simulink model "NatersV4_clean"  (R2016a)
settings: Solver=ode5  StartTime=1  StopTime=12*24*3  FixedStep=1  RelTol=1e-3
InitFcn:
  | %open the initialization function as a structure s
  | clear all
  | model = 'NatersV4_clean';
  | s = system_init(model);
  | clear ans
  | 
  | % time vector
  | t=s.t;
  | t_step = t(2)-t(1);
  | time_u = s.time(1);
  | sample_time = s.sample_time;
  | 
  | % declare parameters
  | building = s.building;
  | Text_D = s.Design(1);
  | Tin_D = s.Design(2);
  | Ts_D = s.Design(3);
  | Tr_D = s.Design(4);
  | Qdot_dem = s.Qdot_dem;
  | L_ini= s.L_ini;
  | 
  | Ab_c = s.Ab_c;
  | Bb_c = s.Bb_c;
  | Tin_sp = s.Tin_sp.signals.values;
  | Text = s.Text.signals.values;
  | Rad_90 = s.rad_90.signals.values;
  | 
  | % k parameters for heat pump model
  | K = s.k;
undefined symbols (not defined in the file or in its folder): DiscIntNeverNeededParam
libraries: simulink x17, carnot x2, dspsigops x1
(part 1 of 2)
settings Model: Creator=frederic.amblard  LastModifiedBy=frederic.amblard
settings DataIOCC: ExternalInput=[t, Ab_c, Bb_c, Text, Tin_sp]

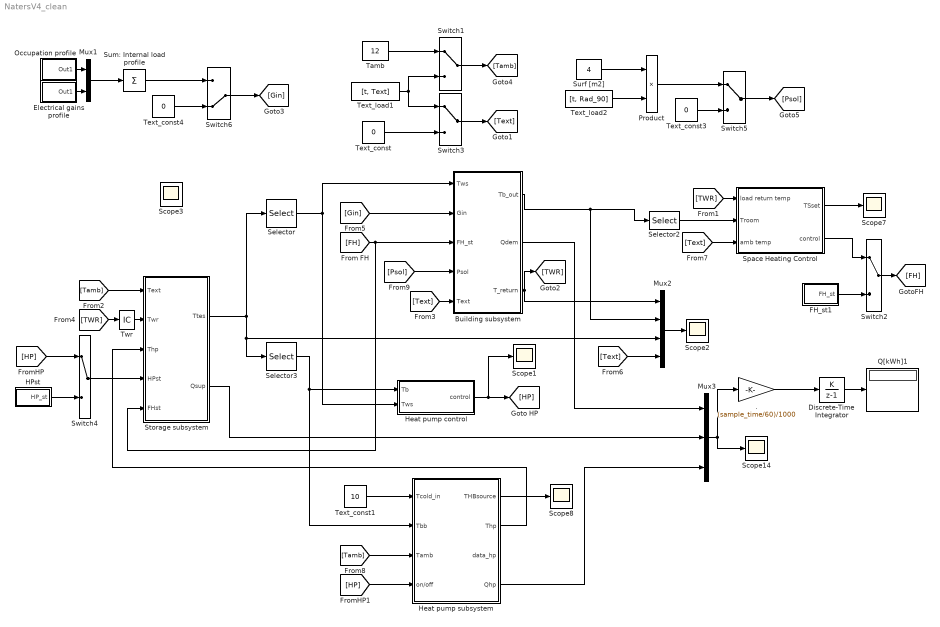
== system NatersV4_clean ==
  . : Gain  Gain=(sample_time/60)/1000  SaturateOnIntegerOverflow=on  OutDataTypeStr=Inherit: Same as input  ParamDataTypeStr=Inherit: Same as input
  Building subsystem : Subsystem
  Discrete-Time Integrator : DiscreteIntegrator  IntegratorMethod=Accumulation: Forward Euler  InitialConditionSetting=State (most efficient)  SampleTime=-1  ICPrevOutput=DiscIntNeverNeededParam  ICPrevScaledInput=DiscIntNeverNeededParam
  Electrical gains profile : Subsystem  mask{period=24*60/sample_time, rep_seq_t=[0 1 6 7 8 9 11 12 13 18 19 20 22 23]*60/sample_time, rep_seq_d=[1 5 1 1 1 2 1 1 4 2 1 2 1 1]*60/sample_time, rep_seq_y=[105 55 392.5 457.5 420 55 250 55 120 170 615 420 442.5 355]*60/sample_time}
      mask prompts: period "Timeperiod in h"; rep_seq_t "Time values in h"; rep_seq_d "Duration in h"; rep_seq_y "Output values"
  FH_st1 : Subsystem  mask{period=24*60/sample_time, rep_seq_t=[0 6 7 8 9 11 12 13 14 15 17 18 20 21 22]*60/sample_time, rep_seq_d=[6 1 1 1 2 1 1 1 1 2 1 2 1 1 2]*60/sample_time, rep_seq_y=[1 1 1 0 0 0 1 1 1 0 0 1 1 1 1]*60/sample_time}
      mask prompts: period "Timeperiod in h"; rep_seq_t "Time values in h"; rep_seq_d "Duration in h"; rep_seq_y "Output values"
  HPst : Subsystem  mask{period=24*60/sample_time, rep_seq_t=[0 6 7 8 9 11 12 13 14 15 17 18 20 21 22]*60/sample_time, rep_seq_d=[6 1 1 1 2 1 1 1 1 2 1 2 1 1 2]*60/sample_time, rep_seq_y=[1 1 1 0 0 0 1 1 1 0 0 1 1 1 1]*60/sample_time}
      mask prompts: period "Timeperiod in h"; rep_seq_t "Time values in h"; rep_seq_d "Duration in h"; rep_seq_y "Output values"
  Heat pump control : Subsystem
  Heat pump subsystem : Subsystem  mask{K=K, caph=80000, capc=50000, cp=4185, DT=4, UA=7, Qdot_D=Qdot_dem}
      mask prompts: K "Param K"; caph "Thermal capacity hot side [J/K]"; capc "Thermal capacity cold side [J/K]"; cp "Heat capacity of water [J/(kg·K)]"; DT "Delta temperature fixed cold side"; UA "Heat loss coefficient [W/K]"; Qdot_D "Design thermal power [W]"
      mask init:
      | mcdot = 1000*Qdot_D/(DT*cp) / 1000; % mass flow [kg/s]
  Mux1 : Mux  Inputs=2
  Mux2 : Mux
  Mux3 : Mux  Inputs=3
  Occupation profile : Subsystem  mask{period=24*60/sample_time, rep_seq_t=[0 6 7 8 9 11 12 13 14 15 17 18 20 21 22]*60/sample_time, rep_seq_d=[6 1 1 1 2 1 1 1 1 2 1 2 1 1 2]*60/sample_time, rep_seq_y=[4 2 3 2 0 1 3 2 1 0 1 2 4 3 4]*60*60/sample_time}
      mask prompts: period "Timeperiod in h"; rep_seq_t "Time values in h"; rep_seq_d "Duration in h"; rep_seq_y "Output values"
  Product : Product
  Q[kWh]1 : Display
  Scope{1..3,7..8,14} (6 alike) : Scope
  Selector : Selector  InputPortWidth=3  IndexOptions=Index vector (dialog)  Indices=[1]  OutputSizes=1
  Selector2 : Selector  InputPortWidth=2  IndexOptions=Index vector (dialog)  Indices=[2]  OutputSizes=1
  Selector3 : Selector  InputPortWidth=3  IndexOptions=Index vector (dialog)  Indices=[3]  OutputSizes=1
  Space Heating Control : Subsystem  mask{Tset=Tin_D, Tsetn=Tin_D, Q_LOC=Qdot_dem, Td_in=Ts_D, Td_out=Tr_D, Tambd=Text_D, n_rad=1.1}
      mask prompts: Tset "desired room day Temperature [°C]"; Tsetn "desired room night Temperature [°C]"; Q_LOC "design heat load [W]"; Td_in "design inlet temperature of the heating system [°C]"; Td_out "design outlet temperature of the heating system [°C]"; Tambd "design outdoor temperature"; n_rad "radiatior exponent"
      mask init:
      | dTd = 0.5*(Td_in + Td_out) - Tset;
      | dTdn = 0.5*(Td_in + Td_out) - Tsetn;
  Storage subsystem : Subsystem
  Sum: Internal load profile : Sum  Inputs=+
  Surf [m2] : Constant  Value=4
  Switch{1..5} (5 alike) : ManualSwitch
  Switch6 : ManualSwitch  CurrentSetting=0
  Tamb : Constant  Value=12
  Text_const : Constant  Value=0
  Text_const1 : Constant  Value=10
  Text_const3 : Constant  Value=0
  Text_const4 : Constant  Value=0
  Text_load1 : FromWorkspace  Tag=Tin_sp  Description=Temperature signal of the room  VariableName=[t, Text]  SampleTime=1  Interpolate=off  OutputAfterFinalValue=Setting to zero
  Text_load2 : FromWorkspace  Tag=Tin_sp  Description=Temperature signal of the room  VariableName=[t, Rad_90]  SampleTime=1  Interpolate=off  OutputAfterFinalValue=Setting to zero
  Twr : InitialCondition  Value=Tr_D
  wires:
  Text_load1/1 -> Switch1/2, Switch3/1
  Text_const/1 -> Switch3/2
  Switch3/1 -> [Text]
  [Tamb] -> Storage subsystem/1(Text)
  Storage subsystem/1(Ttes) -> Selector/1, Selector3/1, Mux2/3
  Occupation profile/1(Out1) -> Mux1/1
  Electrical gains profile/1(Out1) -> Mux1/2
  Mux1/1 -> Sum: Internal load profile/1
  Sum: Internal load profile/1 -> Switch6/1
  Building subsystem/1(Tb_out) -> Mux2/2, Selector2/1
  Building subsystem/3(T_return) -> Mux2/1, [TWR]
  [TWR] -> Twr/1
  Twr/1 -> Storage subsystem/2(Twr)
  [Gin] -> Building subsystem/2(Gin)
  Text_load2/1 -> Product/2
  Mux2/1 -> Scope2/1
  HPst/1(HP_st) -> Switch4/2
  [Text] -> Mux2/4
  Tamb/1 -> Switch1/1
  Switch1/1 -> [Tamb]
  [FH] -> Storage subsystem/5(FHst), Building subsystem/3(FH_st)
  Selector2/1 -> Space Heating Control/2(Troom)
  [Text] -> Space Heating Control/3(amb temp)
  Space Heating Control/1(TSset) -> Scope7/1
  Space Heating Control/2(control) -> Switch2/1
  FH_st1/1(FH_st) -> Switch2/2
  Switch2/1 -> [FH]
  Switch4/1 -> Storage subsystem/4(HPst)
  [HP] -> Switch4/1
  Selector3/1 -> Heat pump subsystem/2(Tbb), Heat pump control/1(Tb)
  [Tamb] -> Heat pump subsystem/3(Tamb)
  [HP] -> Heat pump subsystem/4(on/off)
  Heat pump subsystem/1(THBsource) -> Scope8/1
  Heat pump subsystem/2(Thp) -> Storage subsystem/3(Thp)
  Text_const1/1 -> Heat pump subsystem/1(Tcold_in)
  Surf [m2]/1 -> Product/1
  Product/1 -> Switch5/1
  [Psol] -> Building subsystem/4(Psol)
  Storage subsystem/2(Qsup) -> Mux3/2
  Building subsystem/2(Qdem) -> Mux3/1
  Selector/1 -> Heat pump control/2(Tws), Building subsystem/1(Tws)
  Mux3/1 -> Scope14/1, ./1
  Discrete-Time Integrator/1 -> Q[kWh]1/1
  ./1 -> Discrete-Time Integrator/1
  Text_const3/1 -> Switch5/2
  Switch5/1 -> [Psol]
  Text_const4/1 -> Switch6/2
  Switch6/1 -> [Gin]
  Heat pump subsystem/4(Qhp) -> Mux3/3
  [Text] -> Building subsystem/5(Text)
  Heat pump control/1(control) -> Scope1/1, [HP]
  [TWR] -> Space Heating Control/1(load return temp)

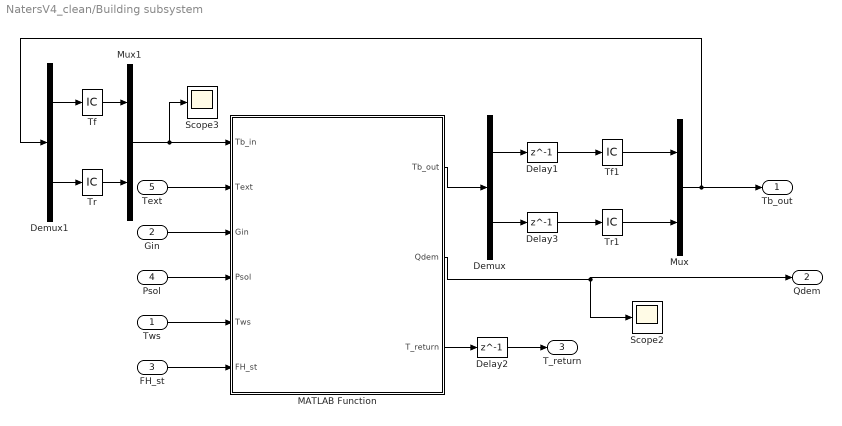
== system NatersV4_clean/Building subsystem ==
  Tws : Inport
  Gin : Inport  Port=2
  FH_st : Inport  Port=3
  Psol : Inport  Port=4
  Text : Inport  Port=5
  Delay1 : Delay  DelayLength=1  InitialCondition=0
  Delay2 : Delay  DelayLength=1  InitialCondition=0
  Delay3 : Delay  DelayLength=1  InitialCondition=0
  Demux : Demux  Outputs=2
  Demux1 : Demux  Outputs=2
  MATLAB Function : MATLAB Function  TreatAsAtomicUnit=on  mask{t_step=t_step, time_u=time_u}
      mask prompts: t_step "time_sample"; time_u "time_unit"
  Mux : Mux  Inputs=2
  Mux1 : Mux  Inputs=2
  Scope2 : Scope
  Scope3 : Scope
  Tf : InitialCondition  Value=22
  Tf1 : InitialCondition  Value=22
  Tr : InitialCondition  Value=20
  Tr1 : InitialCondition  Value=20
  Tb_out : Outport
  Qdem : Outport  Port=2
  T_return : Outport  Port=3
  wires:
  MATLAB Function/1(Tb_out) -> Demux/1
  Delay1/1 -> Tf1/1
  Delay3/1 -> Tr1/1
  Demux/1 -> Delay1/1
  Demux/2 -> Delay3/1
  Mux/1 -> Demux1/1, Tb_out/1
  Tr/1 -> Mux1/2
  Demux1/2 -> Tr/1
  Demux1/1 -> Tf/1
  Tf/1 -> Mux1/1
  Mux1/1 -> Scope3/1, MATLAB Function/1(Tb_in)
  FH_st/1 -> MATLAB Function/6(FH_st)
  Gin/1 -> MATLAB Function/3(Gin)
  Psol/1 -> MATLAB Function/4(Psol)
  MATLAB Function/2(Qdem) -> Scope2/1, Qdem/1
  Tws/1 -> MATLAB Function/5(Tws)
  Text/1 -> MATLAB Function/2(Text)
  Tf1/1 -> Mux/1
  Tr1/1 -> Mux/2
  MATLAB Function/3(T_return) -> Delay2/1
  Delay2/1 -> T_return/1

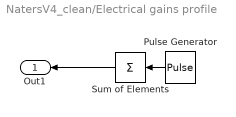
== system NatersV4_clean/Electrical gains profile ==
  Pulse Generator : DiscretePulseGenerator  PulseType=Time based  Amplitude=rep_seq_y  Period=period  PulseWidth=rep_seq_d*100/period  PhaseDelay=rep_seq_t
  Sum of Elements : Sum  Inputs=+
  Out1 : Outport
  wires:
  Sum of Elements/1 -> Out1/1
  Pulse Generator/1 -> Sum of Elements/1

== system NatersV4_clean/FH_st1 ==
  Pulse Generator : DiscretePulseGenerator  PulseType=Time based  Amplitude=rep_seq_y  Period=period  PulseWidth=rep_seq_d*100/period  PhaseDelay=rep_seq_t
  Sum of Elements : Sum  Inputs=+
  FH_st : Outport
  wires:
  Sum of Elements/1 -> FH_st/1
  Pulse Generator/1 -> Sum of Elements/1

== system NatersV4_clean/HPst ==
  Pulse Generator : DiscretePulseGenerator  PulseType=Time based  Amplitude=rep_seq_y  Period=period  PulseWidth=rep_seq_d*100/period  PhaseDelay=rep_seq_t
  Sum of Elements : Sum  Inputs=+
  HP_st : Outport
  wires:
  Sum of Elements/1 -> HP_st/1
  Pulse Generator/1 -> Sum of Elements/1

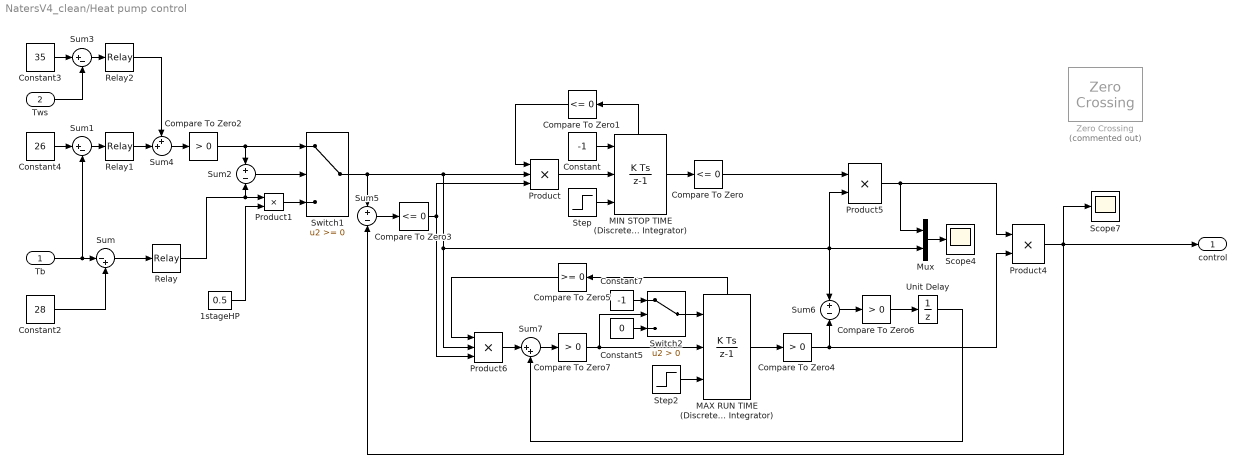
== system NatersV4_clean/Heat pump control ==
  Tb : Inport
  Tws : Inport  Port=2
  1stageHP : Constant  Value=0.5
  Compare To Zero : simulink/Logic and Bit Operations/Compare To Zero  relop=<=  OutDataTypeStr=uint8
  Compare To Zero1 : simulink/Logic and Bit Operations/Compare To Zero  relop=<=  OutDataTypeStr=uint8
  Compare To Zero2 : simulink/Logic and Bit Operations/Compare To Zero  relop=>  OutDataTypeStr=boolean
  Compare To Zero3 : simulink/Logic and Bit Operations/Compare To Zero  relop=<=  OutDataTypeStr=uint8
  Compare To Zero4 : simulink/Logic and Bit Operations/Compare To Zero  relop=>  OutDataTypeStr=uint8
  Compare To Zero5 : simulink/Logic and Bit Operations/Compare To Zero  relop=>=  OutDataTypeStr=uint8
  Compare To Zero6 : simulink/Logic and Bit Operations/Compare To Zero  relop=>  OutDataTypeStr=uint8
  Compare To Zero7 : simulink/Logic and Bit Operations/Compare To Zero  relop=>  OutDataTypeStr=uint8
  Constant : Constant  Value=-1
  Constant2 : Constant  Value=28
  Constant3 : Constant  Value=35
  Constant4 : Constant  Value=26
  Constant5 : Constant  Value=0  SampleTime=-1
  Constant7 : Constant  Value=-1  SampleTime=-1
  MAX RUN TIME (Discrete-Time Integrator) : DiscreteIntegrator  ExternalReset=falling  InitialConditionSource=external  InitialConditionSetting=State (most efficient)  SampleTime=-1  LowerSaturationLimit=0  ShowStatePort=on  IgnoreLimit=on  ICPrevOutput=DiscIntNeverNeededParam  ICPrevScaledInput=DiscIntNeverNeededParam
  MIN STOP TIME (Discrete-Time Integrator) : DiscreteIntegrator  ExternalReset=falling  InitialConditionSource=external  InitialConditionSetting=State (most efficient)  SampleTime=-1  LimitOutput=on  LowerSaturationLimit=0  ShowStatePort=on  ICPrevOutput=DiscIntNeverNeededParam  ICPrevScaledInput=DiscIntNeverNeededParam
  Mux : Mux  Inputs=2
  Product : Product  Inputs=3  RndMeth=Zero
  Product1 : Product  RndMeth=Zero
  Product4 : Product  RndMeth=Zero
  Product5 : Product  RndMeth=Zero
  Product6 : Product  Inputs=3  RndMeth=Zero
  Relay : Relay  OnSwitchValue=1  OffSwitchValue=-6
  Relay1 : Relay  OnSwitchValue=1  OffSwitchValue=-2
  Relay2 : Relay  OnSwitchValue=1  OffSwitchValue=-6
  Scope4 : Scope
  Scope7 : Scope
  Step : Step  After=15/sample_time  SampleTime=1
  Step2 : Step  After=300/sample_time  SampleTime=1  VectorParams1D=off
  Sum : Sum  Inputs=|-+
  Sum1 : Sum  Inputs=|+-
  Sum2 : Sum  Inputs=+|-
  Sum3 : Sum  Inputs=|+-
  Sum4 : Sum  Inputs=++|
  Sum5 : Sum  Inputs=+|-
  Sum6 : Sum  Inputs=+|-
  Sum7 : Sum  Inputs=|++
  Switch1 : Switch
  Switch2 : Switch  Criteria=u2 > Threshold
  Unit Delay : UnitDelay  SampleTime=-1
  Zero Crossing : dspsigops/Zero Crossing  Commented=on  InputProcessing=Columns as channels (frame based)
  control : Outport
  wires:
  Tb/1 -> Sum/1, Sum1/2
  Constant2/1 -> Sum/2
  Sum/1 -> Relay/1
  Product/1 -> MIN STOP TIME (Discrete-Time Integrator)/2
  MIN STOP TIME (Discrete-Time Integrator)/State -> Compare To Zero1/1
  Compare To Zero1/1 -> Product/1
  Constant/1 -> MIN STOP TIME (Discrete-Time Integrator)/1
  Step/1 -> MIN STOP TIME (Discrete-Time Integrator)/3
  MIN STOP TIME (Discrete-Time Integrator)/1 -> Compare To Zero/1
  Mux/1 -> Scope4/1
  Compare To Zero/1 -> Product5/1
  Product5/1 -> Mux/1, Product4/1
  MAX RUN TIME (Discrete-Time Integrator)/State -> Compare To Zero5/1
  Step2/1 -> MAX RUN TIME (Discrete-Time Integrator)/3
  Relay/1 -> Product1/1, Sum2/2
  1stageHP/1 -> Product1/2
  Constant4/1 -> Sum1/1
  Sum1/1 -> Relay1/1
  Sum4/1 -> Compare To Zero2/1
  Product1/1 -> Switch1/3
  Sum2/1 -> Switch1/2
  Constant3/1 -> Sum3/1
  Tws/1 -> Sum3/2
  Sum3/1 -> Relay2/1
  Relay2/1 -> Sum4/1
  Relay1/1 -> Sum4/2
  Product4/1 -> control/1, Scope7/1, Sum5/2
  Compare To Zero2/1 -> Switch1/1, Sum2/1
  Switch1/1 -> Product/2, Product6/2, Product5/2, Mux/2, Sum6/1, Sum5/1
  Sum5/1 -> Compare To Zero3/1
  Sum6/1 -> Compare To Zero6/1
  Product6/1 -> Sum7/1
  Compare To Zero6/1 -> Unit Delay/1
  Compare To Zero4/1 -> Sum6/2, Product4/2
  Compare To Zero3/1 -> Product/3, Product6/3
  Sum7/1 -> Compare To Zero7/1
  Compare To Zero7/1 -> Switch2/2, MAX RUN TIME (Discrete-Time Integrator)/2
  Unit Delay/1 -> Sum7/2
  Constant7/1 -> Switch2/1
  Compare To Zero5/1 -> Product6/1
  MAX RUN TIME (Discrete-Time Integrator)/1 -> Compare To Zero4/1
  Switch2/1 -> MAX RUN TIME (Discrete-Time Integrator)/1
  Constant5/1 -> Switch2/3

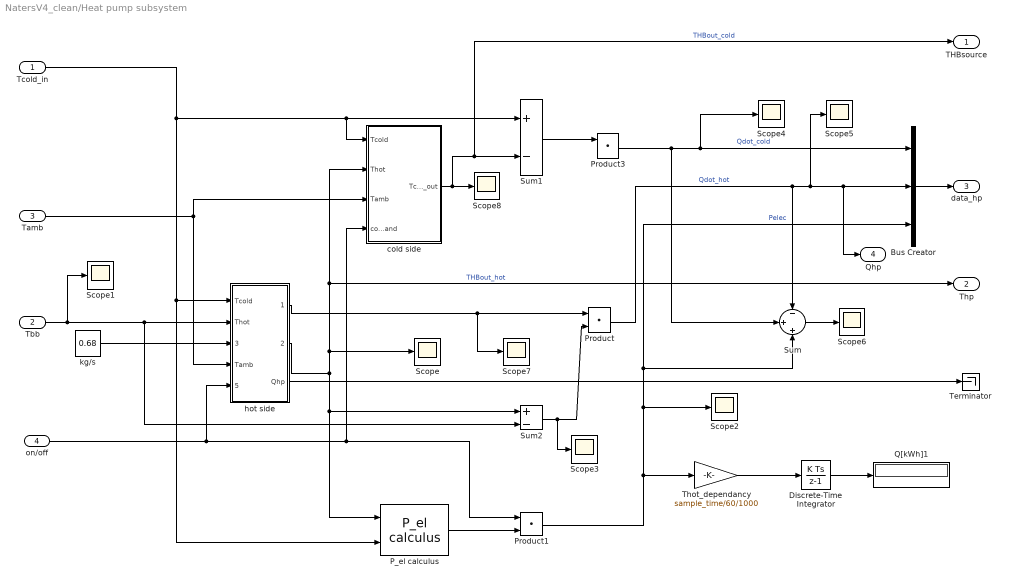
== system NatersV4_clean/Heat pump subsystem ==
  Tcold_in : Inport
  Tbb : Inport  Port=2
  Tamb : Inport  Port=3
  on/off : Inport  Port=4
  Bus Creator : BusCreator  Inputs=3
  Discrete-Time Integrator : DiscreteIntegrator  InitialConditionSetting=State (most efficient)  SampleTime=-1  ICPrevOutput=DiscIntNeverNeededParam  ICPrevScaledInput=DiscIntNeverNeededParam
  P_el calculus : carnot/Basic/Thermal_Models/HeatPump_basic/P_el calculus
  Product : DotProduct  InputSameDT=on  OutDataTypeStr=Inherit: Inherit via internal rule
  Product1 : DotProduct  InputSameDT=on  OutDataTypeStr=Inherit: Inherit via internal rule
  Product3 : DotProduct  InputSameDT=on  OutDataTypeStr=Inherit: Inherit via internal rule
  Q[kWh]1 : Display
  Scope{,1..8} (9 alike) : Scope
  Sum : Sum  Inputs=-|+|+
  Sum1 : Sum  Inputs=+-  SaturateOnIntegerOverflow=on  InputSameDT=on  OutDataTypeStr=Inherit: Same as first input
  Sum2 : Sum  Inputs=+-  SaturateOnIntegerOverflow=on  InputSameDT=on  OutDataTypeStr=Inherit: Same as first input
  Terminator : Terminator
  Thot_dependancy : Gain  Gain=sample_time/60/1000  SaturateOnIntegerOverflow=on  OutDataTypeStr=Inherit: Same as input  ParamDataTypeStr=Inherit: Same as input
  cold side : Subsystem
  hot side : Subsystem
  kg/s : Constant  Value=0.68
  THBsource : Outport
  Thp : Outport  Port=2
  data_hp : Outport  Port=3
  Qhp : Outport  Port=4
  wires:
  Bus Creator/1 -> data_hp/1
  cold side/1(Tcold_out) -> THBsource/1, Sum1/2, Scope8/1  "THBout_cold"
  hot side/2(Thot_out) -> cold side/2(Thot), Thp/1, Scope/1, P_el calculus/1, Sum2/1  "THBout_hot"
  Tamb/1 -> cold side/3(Tamb), hot side/4(Tamb)
  Tbb/1 -> Scope1/1, hot side/2(Thot), Sum2/2
  hot side/1(mdot*cp) -> Scope7/1, Product/1
  Sum2/1 -> Scope3/1, Product/2
  Tcold_in/1 -> hot side/1(Tcold), P_el calculus/2, cold side/1(Tcold), Sum1/1
  P_el calculus/1 -> Product1/2
  Product1/1 -> Thot_dependancy/1, Scope2/1, Sum/3, Bus Creator/3  "Pelec"
  on/off/1 -> hot side/5(command), cold side/4(command), Product1/1
  Sum1/1 -> Product3/1
  Product3/1 -> Sum/2, Scope4/1, Bus Creator/1  "Qdot_cold"
  Product/1 -> Sum/1, Scope5/1, Qhp/1, Bus Creator/2  "Qdot_hot"
  kg/s/1 -> hot side/3(mdot_hot)
  Discrete-Time Integrator/1 -> Q[kWh]1/1
  Thot_dependancy/1 -> Discrete-Time Integrator/1
  Sum/1 -> Scope6/1
  hot side/3(Qhp) -> Terminator/1

== system NatersV4_clean/Occupation profile ==
  Pulse Generator : DiscretePulseGenerator  PulseType=Time based  Amplitude=rep_seq_y  Period=period  PulseWidth=rep_seq_d*100/period  PhaseDelay=rep_seq_t
  Sum of Elements : Sum  Inputs=+
  Out1 : Outport
  wires:
  Sum of Elements/1 -> Out1/1
  Pulse Generator/1 -> Sum of Elements/1

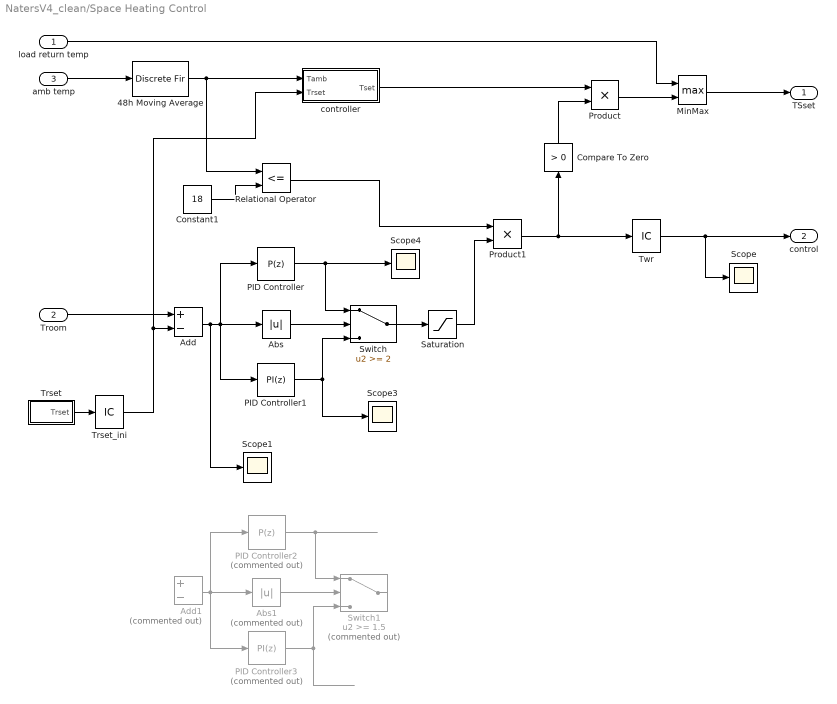
== system NatersV4_clean/Space Heating Control ==
  load return temp : Inport
  Troom : Inport  Port=2
  amb temp : Inport  Port=3
  48h Moving Average : DiscreteFir  Coefficients=ones(1,60/sample_time*24)*(1/((60/sample_time)*24))  SampleTime=1  AccumDataTypeStr=Inherit: Same as product output  RndMeth=Nearest
  Abs : Abs
  Abs1 : Abs  Commented=on
  Add : Sum  Inputs=+-
  Add1 : Sum  Commented=on  Inputs=+-
  Compare To Zero : simulink/Logic and Bit Operations/Compare To Zero  relop=>  OutDataTypeStr=boolean
  Constant1 : Constant  Value=18
  MinMax : MinMax  Function=max  Inputs=2
  PID Controller : simulink/Continuous/PID Controller  Controller=P  TimeDomain=Discrete-time  SampleTime=-1  IntegratorMethod=Forward Euler  FilterMethod=Forward Euler  Form=Parallel  UseFilter=on  ControllerParametersSource=internal  P=-0.6  I=1  D=0  N=100  InitialConditionSource=internal  InitialConditionForIntegrator=0  InitialConditionForFilter=0  ExternalReset=none  ZeroCross=off  LimitOutput=on  UpperSaturationLimit=1  LowerSaturationLimit=0  LinearizeAsGain=off  AntiWindupMode=none  Kb=1  TrackingMode=off  Kt=1  PParamMin=[]  PParamMax=[]  IParamMin=[]  IParamMax=[]  DParamMin=[]  DParamMax=[]  NParamMin=[]  NParamMax=[]  KbParamMin=[]  KbParamMax=[]  KtParamMin=[]  KtParamMax=[]  POutMin=[]  POutMax=[]  IOutMin=[]  IOutMax=[]  DOutMin=[]  DOutMax=[]  NOutMin=[]  NOutMax=[]  KbOutMin=[]  KbOutMax=[]  KtOutMin=[]  KtOutMax=[]  IntegratorOutMin=[]  IntegratorOutMax=[]  FilterOutMin=[]  FilterOutMax=[]  SumOutMin=[]  SumOutMax=[]  SumI1OutMin=[]  SumI1OutMax=[]  SumI2OutMin=[]  SumI2OutMax=[]  SumI3OutMin=[]  SumI3OutMax=[]  SumDOutMin=[]  SumDOutMax=[]  SaturationOutMin=[]  SaturationOutMax=[]  IntegratorContinuousStateAttributes=''  IntegratorStateMustResolveToSignalObject=off  IntegratorRTWStateStorageClass=Auto  FilterContinuousStateAttributes=''  FilterStateMustResolveToSignalObject=off  FilterRTWStateStorageClass=Auto  DifferentiatorICPrevScaledInput=0  DifferentiatorOutMin=[]  DifferentiatorOutMax=[]
  PID Controller1 : simulink/Continuous/PID Controller  Controller=PI  TimeDomain=Discrete-time  SampleTime=-1  IntegratorMethod=Trapezoidal  FilterMethod=Forward Euler  Form=Parallel  UseFilter=on  ControllerParametersSource=internal  P=-8  I=-0.8/(60*sample_time)  D=0.001  N=100  InitialConditionSource=internal  InitialConditionForIntegrator=0  InitialConditionForFilter=0  ExternalReset=none  LimitOutput=on  UpperSaturationLimit=1  LowerSaturationLimit=0  LinearizeAsGain=off  AntiWindupMode=back-calculation  Kb=1  TrackingMode=off  Kt=1  PParamMin=[]  PParamMax=[]  IParamMin=[]  IParamMax=[]  DParamMin=[]  DParamMax=[]  NParamMin=[]  NParamMax=[]  KbParamMin=[]  KbParamMax=[]  KtParamMin=[]  KtParamMax=[]  POutMin=[]  POutMax=[]  IOutMin=[]  IOutMax=[]  DOutMin=[]  DOutMax=[]  NOutMin=[]  NOutMax=[]  KbOutMin=[]  KbOutMax=[]  KtOutMin=[]  KtOutMax=[]  IntegratorOutMin=[]  IntegratorOutMax=[]  FilterOutMin=[]  FilterOutMax=[]  SumOutMin=[]  SumOutMax=[]  SumI1OutMin=[]  SumI1OutMax=[]  SumI2OutMin=[]  SumI2OutMax=[]  SumI3OutMin=[]  SumI3OutMax=[]  SumDOutMin=[]  SumDOutMax=[]  SaturationOutMin=[]  SaturationOutMax=[]  IntegratorContinuousStateAttributes=''  IntegratorStateMustResolveToSignalObject=off  IntegratorRTWStateStorageClass=Auto  FilterContinuousStateAttributes=''  FilterStateMustResolveToSignalObject=off  FilterRTWStateStorageClass=Auto  DifferentiatorICPrevScaledInput=0  DifferentiatorOutMin=[]  DifferentiatorOutMax=[]
  PID Controller2 : simulink/Continuous/PID Controller  Commented=on  Controller=P  TimeDomain=Discrete-time  SampleTime=-1  IntegratorMethod=Forward Euler  FilterMethod=Forward Euler  Form=Parallel  UseFilter=on  ControllerParametersSource=internal  P=-0.5  I=1  D=0  N=100  InitialConditionSource=internal  InitialConditionForIntegrator=0  InitialConditionForFilter=0  ExternalReset=none  ZeroCross=off  LimitOutput=on  UpperSaturationLimit=1  LowerSaturationLimit=0  LinearizeAsGain=off  AntiWindupMode=none  Kb=1  TrackingMode=off  Kt=1  PParamMin=[]  PParamMax=[]  IParamMin=[]  IParamMax=[]  DParamMin=[]  DParamMax=[]  NParamMin=[]  NParamMax=[]  KbParamMin=[]  KbParamMax=[]  KtParamMin=[]  KtParamMax=[]  POutMin=[]  POutMax=[]  IOutMin=[]  IOutMax=[]  DOutMin=[]  DOutMax=[]  NOutMin=[]  NOutMax=[]  KbOutMin=[]  KbOutMax=[]  KtOutMin=[]  KtOutMax=[]  IntegratorOutMin=[]  IntegratorOutMax=[]  FilterOutMin=[]  FilterOutMax=[]  SumOutMin=[]  SumOutMax=[]  SumI1OutMin=[]  SumI1OutMax=[]  SumI2OutMin=[]  SumI2OutMax=[]  SumI3OutMin=[]  SumI3OutMax=[]  SumDOutMin=[]  SumDOutMax=[]  SaturationOutMin=[]  SaturationOutMax=[]  IntegratorContinuousStateAttributes=''  IntegratorStateMustResolveToSignalObject=off  IntegratorRTWStateStorageClass=Auto  FilterContinuousStateAttributes=''  FilterStateMustResolveToSignalObject=off  FilterRTWStateStorageClass=Auto  DifferentiatorICPrevScaledInput=0  DifferentiatorOutMin=[]  DifferentiatorOutMax=[]
  PID Controller3 : simulink/Continuous/PID Controller  Commented=on  Controller=PI  TimeDomain=Discrete-time  SampleTime=-1  IntegratorMethod=Backward Euler  FilterMethod=Forward Euler  Form=Parallel  UseFilter=on  ControllerParametersSource=internal  P=-0.6  I=-0.05/(60*sample_time)  D=0.001  N=100  InitialConditionSource=internal  InitialConditionForIntegrator=0  InitialConditionForFilter=0  ExternalReset=none  ZeroCross=off  LimitOutput=on  UpperSaturationLimit=1  LowerSaturationLimit=0  LinearizeAsGain=off  AntiWindupMode=back-calculation  Kb=1  TrackingMode=off  Kt=1  PParamMin=[]  PParamMax=[]  IParamMin=[]  IParamMax=[]  DParamMin=[]  DParamMax=[]  NParamMin=[]  NParamMax=[]  KbParamMin=[]  KbParamMax=[]  KtParamMin=[]  KtParamMax=[]  POutMin=[]  POutMax=[]  IOutMin=[]  IOutMax=[]  DOutMin=[]  DOutMax=[]  NOutMin=[]  NOutMax=[]  KbOutMin=[]  KbOutMax=[]  KtOutMin=[]  KtOutMax=[]  IntegratorOutMin=[]  IntegratorOutMax=[]  FilterOutMin=[]  FilterOutMax=[]  SumOutMin=[]  SumOutMax=[]  SumI1OutMin=[]  SumI1OutMax=[]  SumI2OutMin=[]  SumI2OutMax=[]  SumI3OutMin=[]  SumI3OutMax=[]  SumDOutMin=[]  SumDOutMax=[]  SaturationOutMin=[]  SaturationOutMax=[]  IntegratorContinuousStateAttributes=''  IntegratorStateMustResolveToSignalObject=off  IntegratorRTWStateStorageClass=Auto  FilterContinuousStateAttributes=''  FilterStateMustResolveToSignalObject=off  FilterRTWStateStorageClass=Auto  DifferentiatorICPrevScaledInput=0  DifferentiatorOutMin=[]  DifferentiatorOutMax=[]
  Product : Product
  Product1 : Product
  Relational Operator : RelationalOperator  Operator=<=  OutDataTypeStr=boolean
  Saturation : Saturate  UpperLimit=1  LowerLimit=0  LinearizeAsGain=off  ZeroCross=off
  Scope{,1,3..4} (4 alike) : Scope
  Switch : Switch  Threshold=2
  Switch1 : Switch  Commented=on  Threshold=1.5
  Trset : Subsystem  mask{period=24*60/sample_time, rep_seq_t=[0 7 21]*60/sample_time, rep_seq_d=[7 14 3]*60/sample_time, rep_seq_y=[Tsetn Tset Tsetn]}
      mask prompts: period "Timeperiod in h"; rep_seq_t "Time values in h"; rep_seq_d "Duration in h"; rep_seq_y "Output values"
  Trset_ini : InitialCondition  Value=19.9
  Twr : InitialCondition  Value=L_ini
  controller : Subsystem
  TSset : Outport
  control : Outport  Port=2
  wires:
  amb temp/1 -> 48h Moving Average/1
  Constant1/1 -> Relational Operator/2
  Troom/1 -> Add/1
  Add/1 -> Scope1/1, PID Controller/1, PID Controller1/1, Abs/1
  Abs/1 -> Switch/2
  PID Controller/1 -> Scope4/1, Switch/1
  PID Controller1/1 -> Switch/3, Scope3/1
  Switch/1 -> Saturation/1
  Saturation/1 -> Product1/2
  Product/1 -> MinMax/2
  load return temp/1 -> MinMax/1
  Compare To Zero/1 -> Product/2
  48h Moving Average/1 -> Relational Operator/1, controller/1(Tamb)
  controller/1(Tset) -> Product/1
  Relational Operator/1 -> Product1/1
  MinMax/1 -> TSset/1
  Trset/1(Trset) -> Trset_ini/1
  Product1/1 -> Twr/1, Compare To Zero/1
  Add1/1 -> PID Controller2/1, PID Controller3/1, Abs1/1
  Abs1/1 -> Switch1/2
  PID Controller2/1 -> Switch1/1
  PID Controller3/1 -> Switch1/3
  Twr/1 -> Scope/1, control/1
  Trset_ini/1 -> controller/2(Trset), Add/2

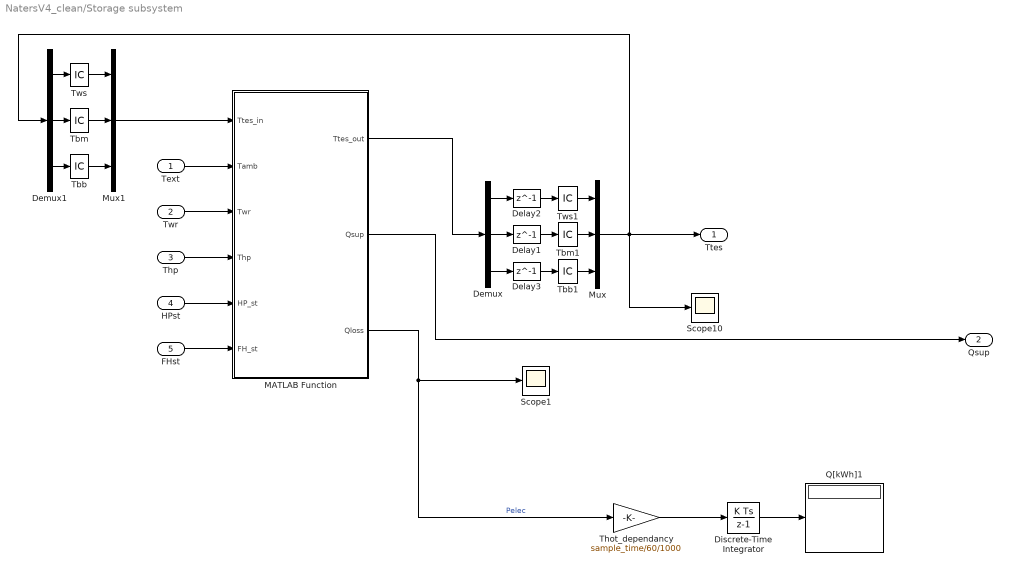
== system NatersV4_clean/Storage subsystem ==
  Text : Inport
  Twr : Inport  Port=2
  Thp : Inport  Port=3
  HPst : Inport  Port=4
  FHst : Inport  Port=5
  Delay1 : Delay  DelayLength=1  InitialCondition=0
  Delay2 : Delay  DelayLength=1  InitialCondition=0
  Delay3 : Delay  DelayLength=1  InitialCondition=0
  Demux : Demux  Outputs=3
  Demux1 : Demux  Outputs=3
  Discrete-Time Integrator : DiscreteIntegrator  InitialConditionSetting=State (most efficient)  SampleTime=-1  ICPrevOutput=DiscIntNeverNeededParam  ICPrevScaledInput=DiscIntNeverNeededParam
  MATLAB Function : MATLAB Function  TreatAsAtomicUnit=on  mask{t_step=t_step, time_u=time_u}
      mask prompts: t_step "sampling_time"; time_u "time_unit"
  Mux : Mux  Inputs=3
  Mux1 : Mux  Inputs=3
  Q[kWh]1 : Display
  Scope1 : Scope
  Scope10 : Scope
  Tbb : InitialCondition  Value=28
  Tbb1 : InitialCondition  Value=28
  Tbm : InitialCondition  Value=31
  Tbm1 : InitialCondition  Value=31
  Thot_dependancy : Gain  Gain=sample_time/60/1000  SaturateOnIntegerOverflow=on  OutDataTypeStr=Inherit: Same as input  ParamDataTypeStr=Inherit: Same as input
  Tws : InitialCondition  Value=35
  Tws1 : InitialCondition  Value=35
  Ttes : Outport
  Qsup : Outport  Port=2
  wires:
  MATLAB Function/1(Ttes_out) -> Demux/1
  Delay2/1 -> Tws1/1
  Delay1/1 -> Tbm1/1
  Text/1 -> MATLAB Function/2(Tamb)
  HPst/1 -> MATLAB Function/5(HP_st)
  FHst/1 -> MATLAB Function/6(FH_st)
  Demux/1 -> Delay2/1
  Demux/2 -> Delay1/1
  Demux1/2 -> Tbm/1
  Tbm/1 -> Mux1/2
  Demux1/1 -> Tws/1
  Tws/1 -> Mux1/1
  Mux1/1 -> MATLAB Function/1(Ttes_in)
  Thp/1 -> MATLAB Function/4(Thp)
  MATLAB Function/2(Qsup) -> Qsup/1
  Twr/1 -> MATLAB Function/3(Twr)
  Discrete-Time Integrator/1 -> Q[kWh]1/1
  Thot_dependancy/1 -> Discrete-Time Integrator/1
  MATLAB Function/3(Qloss) -> Scope1/1, Thot_dependancy/1  "Pelec"
  Demux/3 -> Delay3/1
  Delay3/1 -> Tbb1/1
  Demux1/3 -> Tbb/1
  Tbb/1 -> Mux1/3
  Mux/1 -> Ttes/1, Scope10/1, Demux1/1
  Tws1/1 -> Mux/1
  Tbm1/1 -> Mux/2
  Tbb1/1 -> Mux/3

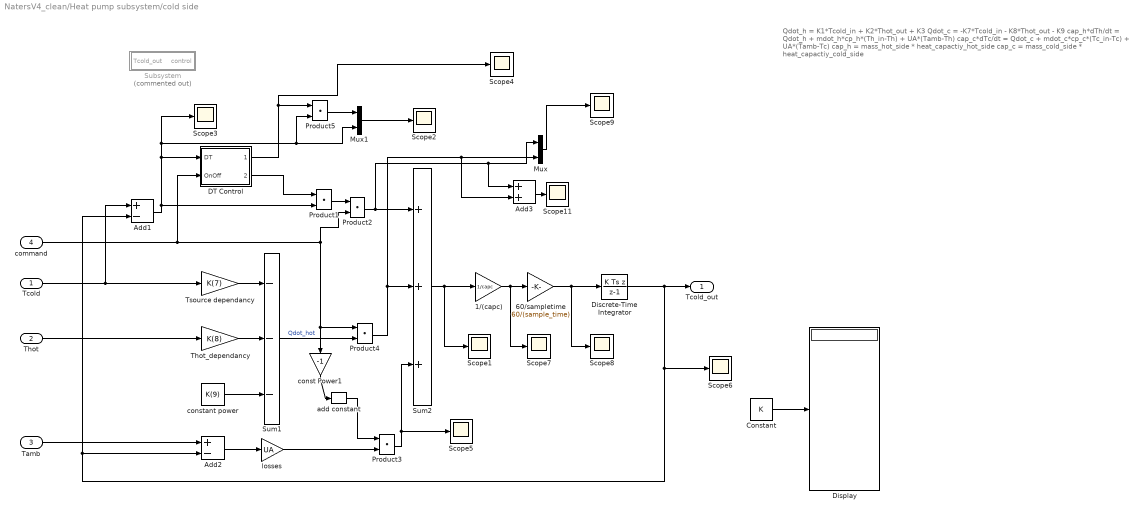
== system NatersV4_clean/Heat pump subsystem/cold side ==
  note: Qdot_h = K1*Tcold_in + K2*Thot_out + K3
      |
      | Qdot_c = -K7*Tcold_in - K8*Thot_out - K9
      |
      | cap_h*dTh/dt = Qdot_h + mdot_h*cp_h*(Th_in-Th) + UA*(Tamb-Th)
      |
      | cap_c*dTc/dt = Qdot_c + mdot_c*cp_c*(Tc_in-Tc) + UA*(Tamb-Tc)
      |
      | cap_h = mass_hot_side * heat_capactiy_hot_side
      |
      | cap_c = mass_cold_side * heat_capactiy_cold_side
  Tcold : Inport
  Thot : Inport  Port=2
  Tamb : Inport  Port=3
  command : Inport  Port=4
  1/(capc) : Gain  Gain=1/capc
  60/sampletime : Gain  Gain=60/(sample_time)
  Add1 : Sum  Inputs=+-
  Add2 : Sum  Inputs=+-
  Add3 : Sum
  Constant : Constant  Value=K
  DT Control : Subsystem  mask{DTset=4, mcdotd=mcdot}
      mask prompts: DTset "Desired delta T on district heating network side"; mcdotd "design mass load on cold side [kg/s]"
  Discrete-Time Integrator : DiscreteIntegrator  IntegratorMethod=Integration: Backward Euler  InitialCondition=4  InitialConditionSetting=State (most efficient)  SampleTime=-1  LimitOutput=on  ICPrevOutput=DiscIntNeverNeededParam  ICPrevScaledInput=DiscIntNeverNeededParam
  Display : Display
  Mux : Mux  Inputs=2
  Mux1 : Mux  Inputs=2
  Product{1..5} (5 alike) : DotProduct  InputSameDT=on  OutDataTypeStr=Inherit: Inherit via internal rule
  Scope{1..9,11} (10 alike) : Scope
  Subsystem : Subsystem  Commented=on
  Sum1 : Sum  Inputs=---  SaturateOnIntegerOverflow=on  InputSameDT=on  OutDataTypeStr=Inherit: Same as first input
  Sum2 : Sum  Inputs=+++  SaturateOnIntegerOverflow=on  InputSameDT=on  OutDataTypeStr=Inherit: Same as first input
  Thot_dependancy : Gain  Gain=K(8)  SaturateOnIntegerOverflow=on  OutDataTypeStr=Inherit: Same as input  ParamDataTypeStr=Inherit: Same as input
  Tsource dependancy : Gain  Gain=K(7)  SaturateOnIntegerOverflow=on  OutDataTypeStr=Inherit: Same as input  ParamDataTypeStr=Inherit: Same as input
  add constant : carnot/Basic/Thermal_Models/HeatPump_basic/model cold side/add constant  c=+1
  const Power1 : Gain  Gain=-1  SaturateOnIntegerOverflow=on  OutDataTypeStr=Inherit: Same as input  ParamDataTypeStr=Inherit: Same as input
  constant power : Constant  Value=K(9)
  losses : Gain  Gain=UA
  Tcold_out : Outport
  wires:
  Product4/1 -> Add3/2, Mux/2, Sum2/2
  Sum2/1 -> 1/(capc)/1, Scope1/1
  const Power1/1 -> add constant/1
  add constant/1 -> Product3/1
  losses/1 -> Product3/2
  command/1 -> Product2/2, const Power1/1, Product4/1, DT Control/2(OnOff)
  Tamb/1 -> Add2/1
  Sum1/1 -> Product4/2  "Qdot_hot"
  constant power/1 -> Sum1/3
  Thot_dependancy/1 -> Sum1/2
  Tsource dependancy/1 -> Sum1/1
  Add2/1 -> losses/1
  Thot/1 -> Thot_dependancy/1
  Constant/1 -> Display/1
  Product3/1 -> Sum2/3, Scope5/1
  1/(capc)/1 -> 60/sampletime/1, Scope7/1
  Discrete-Time Integrator/1 -> Add2/2, Add1/2, Scope6/1, Tcold_out/1
  DT Control/1(control) -> Product5/1, Scope4/1
  Add1/1 -> DT Control/1(DT), Product5/2, Mux1/2, Scope3/1, Product1/2
  Mux/1 -> Scope9/1
  Tcold/1 -> Add1/1, Tsource dependancy/1
  Mux1/1 -> Scope2/1
  Product5/1 -> Mux1/1
  Add3/1 -> Scope11/1
  Product2/1 -> Sum2/1, Add3/1, Mux/1
  DT Control/2(mcdot1) -> Product1/1
  Product1/1 -> Product2/1
  60/sampletime/1 -> Discrete-Time Integrator/1, Scope8/1

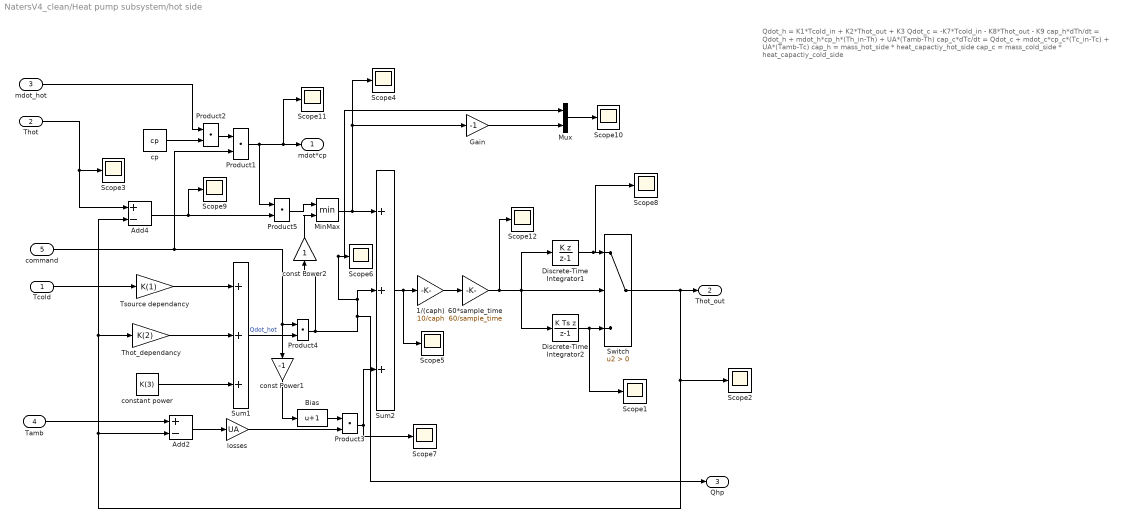
== system NatersV4_clean/Heat pump subsystem/hot side ==
  note: Qdot_h = K1*Tcold_in + K2*Thot_out + K3
      |
      | Qdot_c = -K7*Tcold_in - K8*Thot_out - K9
      |
      | cap_h*dTh/dt = Qdot_h + mdot_h*cp_h*(Th_in-Th) + UA*(Tamb-Th)
      |
      | cap_c*dTc/dt = Qdot_c + mdot_c*cp_c*(Tc_in-Tc) + UA*(Tamb-Tc)
      |
      | cap_h = mass_hot_side * heat_capactiy_hot_side
      |
      | cap_c = mass_cold_side * heat_capactiy_cold_side
  Tcold : Inport
  Thot : Inport  Port=2
  mdot_hot : Inport  Port=3
  Tamb : Inport  Port=4
  command : Inport  Port=5
  1/(caph) : Gain  Gain=10/caph
  60*sample_time : Gain  Gain=60/sample_time
  Add2 : Sum  Inputs=+-
  Add4 : Sum  Inputs=+-
  Bias : Bias  Bias=1
  Discrete-Time Integrator1 : DiscreteIntegrator  IntegratorMethod=Accumulation: Backward Euler  InitialCondition=35  InitialConditionSetting=State (most efficient)  SampleTime=-1  LimitOutput=on  ICPrevOutput=DiscIntNeverNeededParam  ICPrevScaledInput=DiscIntNeverNeededParam
  Discrete-Time Integrator2 : DiscreteIntegrator  IntegratorMethod=Integration: Backward Euler  InitialCondition=35  InitialConditionSetting=State (most efficient)  SampleTime=-1  LimitOutput=on  ICPrevOutput=DiscIntNeverNeededParam  ICPrevScaledInput=DiscIntNeverNeededParam
  Gain : Gain  Gain=-1
  MinMax : MinMax  Inputs=2
  Mux : Mux  Inputs=2
  Product{1..5} (5 alike) : DotProduct  InputSameDT=on  OutDataTypeStr=Inherit: Inherit via internal rule
  Scope{1..12} (12 alike) : Scope
  Sum1 : Sum  Inputs=+++  SaturateOnIntegerOverflow=on  InputSameDT=on  OutDataTypeStr=Inherit: Same as first input
  Sum2 : Sum  Inputs=+++  SaturateOnIntegerOverflow=on  InputSameDT=on  OutDataTypeStr=Inherit: Same as first input
  Switch : Switch  Criteria=u2 > Threshold
  Thot_dependancy : Gain  Gain=K(2)  SaturateOnIntegerOverflow=on  OutDataTypeStr=Inherit: Same as input  ParamDataTypeStr=Inherit: Same as input
  Tsource dependancy : Gain  Gain=K(1)  SaturateOnIntegerOverflow=on  OutDataTypeStr=Inherit: Same as input  ParamDataTypeStr=Inherit: Same as input
  const Power1 : Gain  Gain=-1  SaturateOnIntegerOverflow=on  OutDataTypeStr=Inherit: Same as input  ParamDataTypeStr=Inherit: Same as input
  const Power2 : Gain  SaturateOnIntegerOverflow=on  OutDataTypeStr=Inherit: Same as input  ParamDataTypeStr=Inherit: Same as input
  constant power : Constant  Value=K(3)
  cp : Constant  Value=cp
  losses : Gain  Gain=UA
  mdot*cp : Outport
  Thot_out : Outport  Port=2
  Qhp : Outport  Port=3
  wires:
  Thot/1 -> Add4/1, Scope3/1
  mdot_hot/1 -> Product2/1
  Add2/1 -> losses/1
  Tsource dependancy/1 -> Sum1/1
  Thot_dependancy/1 -> Sum1/2
  constant power/1 -> Sum1/3
  Sum1/1 -> Product4/2  "Qdot_hot"
  Tamb/1 -> Add2/1
  command/1 -> Product1/2, Product4/1, const Power1/1
  losses/1 -> Product3/2
  Bias/1 -> Product3/1
  const Power1/1 -> Bias/1
  Sum2/1 -> Scope5/1, 1/(caph)/1
  Product3/1 -> Scope7/1, Sum2/3
  Product4/1 -> const Power2/1, Qhp/1, Mux/1, Scope6/1, Sum2/2
  cp/1 -> Product2/2
  Tcold/1 -> Tsource dependancy/1
  1/(caph)/1 -> 60*sample_time/1
  Product2/1 -> Product1/1
  Product1/1 -> Scope11/1, mdot*cp/1, Product5/1
  Discrete-Time Integrator2/1 -> Switch/3, Scope1/1
  Discrete-Time Integrator1/1 -> Scope8/1, Switch/1
  Mux/1 -> Scope10/1
  Gain/1 -> Mux/2
  Switch/1 -> Add4/2, Thot_dependancy/1, Add2/2, Scope2/1, Thot_out/1
  60*sample_time/1 -> Scope12/1, Discrete-Time Integrator1/1, Discrete-Time Integrator2/1, Switch/2
  MinMax/1 -> Gain/1, Scope4/1, Sum2/1
  Product5/1 -> MinMax/1
  const Power2/1 -> MinMax/2
  Add4/1 -> Scope9/1, Product5/2

== system NatersV4_clean/Space Heating Control/Trset ==
  Pulse Generator : DiscretePulseGenerator  PulseType=Time based  Amplitude=rep_seq_y  Period=period  PulseWidth=rep_seq_d*100/period  PhaseDelay=rep_seq_t
  Sum of Elements : Sum  Inputs=+
  Trset : Outport
  wires:
  Pulse Generator/1 -> Sum of Elements/1
  Sum of Elements/1 -> Trset/1

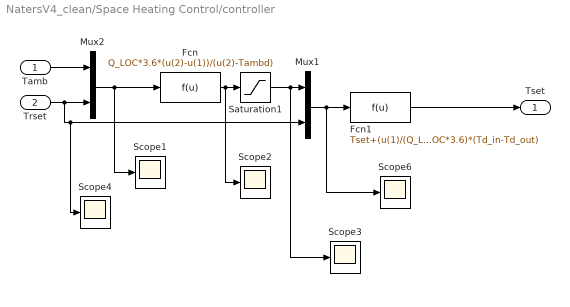
== system NatersV4_clean/Space Heating Control/controller ==
  Tamb : Inport
  Trset : Inport  Port=2
  Fcn : Fcn  Expr=Q_LOC*3.6*(u(2)-u(1))/(u(2)-Tambd)
  Fcn1 : Fcn  Expr=Tset+(u(1)/(Q_LOC*3.6))^(1/n_rad)*(0.5*(Td_in + Td_out) - u(2))+u(1)/(2*Q_LOC*3.6)*(Td_in-Td_out)
  Mux1 : Mux  Inputs=2
  Mux2 : Mux  Inputs=2
  Saturation1 : Saturate  UpperLimit=inf  LowerLimit=0
  Scope{1..4,6} (5 alike) : Scope
  Tset : Outport
  wires:
  Tamb/1 -> Mux2/1
  Fcn/1 -> Scope2/1, Saturation1/1
  Fcn1/1 -> Tset/1
  Saturation1/1 -> Scope3/1, Mux1/1
  Mux2/1 -> Scope1/1, Fcn/1
  Trset/1 -> Scope4/1, Mux1/2, Mux2/2
  Mux1/1 -> Scope6/1, Fcn1/1

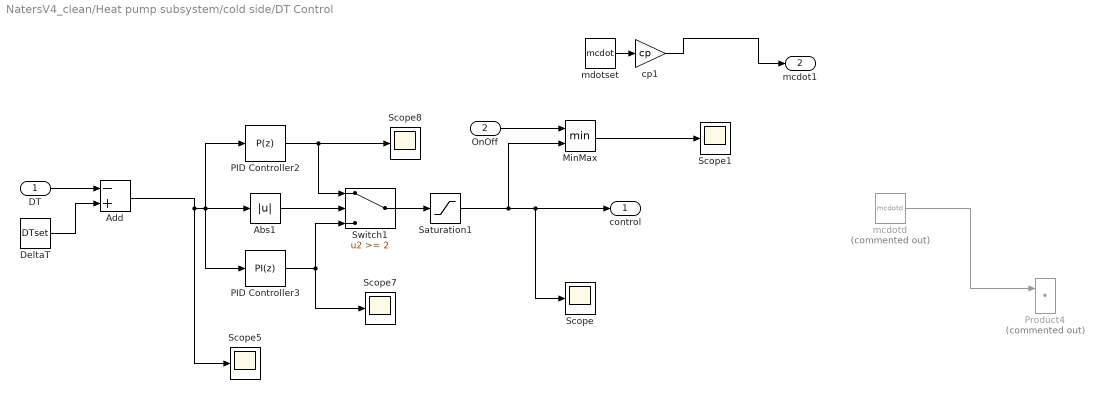
== system NatersV4_clean/Heat pump subsystem/cold side/DT Control ==
  DT : Inport
  OnOff : Inport  Port=2
  Abs1 : Abs
  Add : Sum  Inputs=-+
  DeltaT : Constant  Value=DTset
  MinMax : MinMax  Inputs=2
  PID Controller2 : simulink/Continuous/PID Controller  Controller=P  TimeDomain=Discrete-time  SampleTime=-1  IntegratorMethod=Forward Euler  FilterMethod=Forward Euler  Form=Parallel  UseFilter=on  ControllerParametersSource=internal  P=-4  I=1  D=0  N=100  InitialConditionSource=internal  InitialConditionForIntegrator=0  InitialConditionForFilter=0  ExternalReset=none  ZeroCross=off  LimitOutput=on  UpperSaturationLimit=1  LowerSaturationLimit=0  LinearizeAsGain=off  AntiWindupMode=none  Kb=1  TrackingMode=off  Kt=1  PParamMin=[]  PParamMax=[]  IParamMin=[]  IParamMax=[]  DParamMin=[]  DParamMax=[]  NParamMin=[]  NParamMax=[]  KbParamMin=[]  KbParamMax=[]  KtParamMin=[]  KtParamMax=[]  POutMin=[]  POutMax=[]  IOutMin=[]  IOutMax=[]  DOutMin=[]  DOutMax=[]  NOutMin=[]  NOutMax=[]  KbOutMin=[]  KbOutMax=[]  KtOutMin=[]  KtOutMax=[]  IntegratorOutMin=[]  IntegratorOutMax=[]  FilterOutMin=[]  FilterOutMax=[]  SumOutMin=[]  SumOutMax=[]  SumI1OutMin=[]  SumI1OutMax=[]  SumI2OutMin=[]  SumI2OutMax=[]  SumI3OutMin=[]  SumI3OutMax=[]  SumDOutMin=[]  SumDOutMax=[]  SaturationOutMin=[]  SaturationOutMax=[]  IntegratorContinuousStateAttributes=''  IntegratorStateMustResolveToSignalObject=off  IntegratorRTWStateStorageClass=Auto  FilterContinuousStateAttributes=''  FilterStateMustResolveToSignalObject=off  FilterRTWStateStorageClass=Auto  DifferentiatorICPrevScaledInput=0  DifferentiatorOutMin=[]  DifferentiatorOutMax=[]
  PID Controller3 : simulink/Continuous/PID Controller  Controller=PI  TimeDomain=Discrete-time  SampleTime=-1  IntegratorMethod=Forward Euler  FilterMethod=Forward Euler  Form=Parallel  UseFilter=on  ControllerParametersSource=internal  P=-8  I=-0.2/(60*sample_time)*10  D=0  N=100  InitialConditionSource=internal  InitialConditionForIntegrator=0  InitialConditionForFilter=0  ExternalReset=none  ZeroCross=off  LimitOutput=on  UpperSaturationLimit=1  LowerSaturationLimit=0  LinearizeAsGain=off  AntiWindupMode=back-calculation  Kb=1  TrackingMode=off  Kt=1  PParamMin=[]  PParamMax=[]  IParamMin=[]  IParamMax=[]  DParamMin=[]  DParamMax=[]  NParamMin=[]  NParamMax=[]  KbParamMin=[]  KbParamMax=[]  KtParamMin=[]  KtParamMax=[]  POutMin=[]  POutMax=[]  IOutMin=[]  IOutMax=[]  DOutMin=[]  DOutMax=[]  NOutMin=[]  NOutMax=[]  KbOutMin=[]  KbOutMax=[]  KtOutMin=[]  KtOutMax=[]  IntegratorOutMin=[]  IntegratorOutMax=[]  FilterOutMin=[]  FilterOutMax=[]  SumOutMin=[]  SumOutMax=[]  SumI1OutMin=[]  SumI1OutMax=[]  SumI2OutMin=[]  SumI2OutMax=[]  SumI3OutMin=[]  SumI3OutMax=[]  SumDOutMin=[]  SumDOutMax=[]  SaturationOutMin=[]  SaturationOutMax=[]  IntegratorContinuousStateAttributes=''  IntegratorStateMustResolveToSignalObject=off  IntegratorRTWStateStorageClass=Auto  FilterContinuousStateAttributes=''  FilterStateMustResolveToSignalObject=off  FilterRTWStateStorageClass=Auto  DifferentiatorICPrevScaledInput=0  DifferentiatorOutMin=[]  DifferentiatorOutMax=[]
  Product4 : DotProduct  Commented=on  InputSameDT=on  OutDataTypeStr=Inherit: Inherit via internal rule
  Saturation1 : Saturate  UpperLimit=1  LowerLimit=0  ZeroCross=off
  Scope{,1,5,7..8} (5 alike) : Scope
  Switch1 : Switch  Threshold=2
  cp1 : Gain  Gain=cp  SaturateOnIntegerOverflow=on  OutDataTypeStr=Inherit: Same as input  ParamDataTypeStr=Inherit: Same as input
  mcdotd : Constant  Commented=on  Value=mcdotd
  mdotset : Constant  Value=mcdot
  control : Outport
  mcdot1 : Outport  Port=2
  wires:
  mcdotd/1 -> Product4/1
  DeltaT/1 -> Add/2
  DT/1 -> Add/1
  mdotset/1 -> cp1/1
  cp1/1 -> mcdot1/1
  Add/1 -> Scope5/1, PID Controller2/1, PID Controller3/1, Abs1/1
  Abs1/1 -> Switch1/2
  PID Controller2/1 -> Scope8/1, Switch1/1
  PID Controller3/1 -> Switch1/3, Scope7/1
  Switch1/1 -> Saturation1/1
  Saturation1/1 -> MinMax/2, Scope/1, control/1
  MinMax/1 -> Scope1/1
  OnOff/1 -> MinMax/1

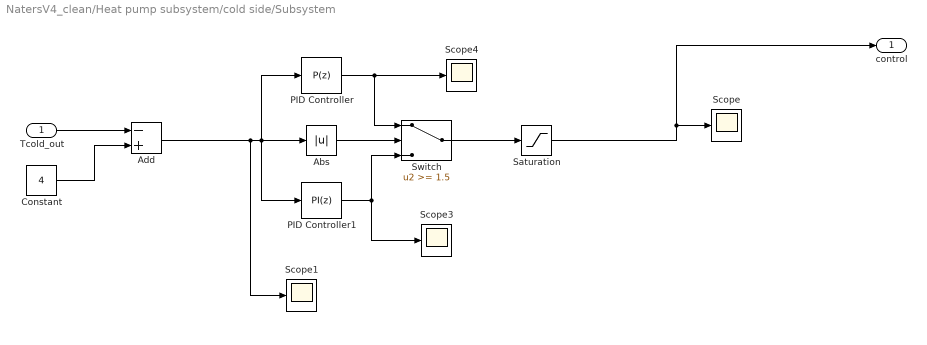
== system NatersV4_clean/Heat pump subsystem/cold side/Subsystem ==
  Tcold_out : Inport
  Abs : Abs
  Add : Sum  Inputs=-+
  Constant : Constant  Value=4
  PID Controller : simulink/Continuous/PID Controller  Controller=P  TimeDomain=Discrete-time  SampleTime=-1  IntegratorMethod=Forward Euler  FilterMethod=Forward Euler  Form=Parallel  UseFilter=on  ControllerParametersSource=internal  P=-0.5  I=1  D=0  N=100  InitialConditionSource=internal  InitialConditionForIntegrator=0  InitialConditionForFilter=0  ExternalReset=none  ZeroCross=off  LimitOutput=on  UpperSaturationLimit=1  LowerSaturationLimit=0  LinearizeAsGain=off  AntiWindupMode=none  Kb=1  TrackingMode=off  Kt=1  PParamMin=[]  PParamMax=[]  IParamMin=[]  IParamMax=[]  DParamMin=[]  DParamMax=[]  NParamMin=[]  NParamMax=[]  KbParamMin=[]  KbParamMax=[]  KtParamMin=[]  KtParamMax=[]  POutMin=[]  POutMax=[]  IOutMin=[]  IOutMax=[]  DOutMin=[]  DOutMax=[]  NOutMin=[]  NOutMax=[]  KbOutMin=[]  KbOutMax=[]  KtOutMin=[]  KtOutMax=[]  IntegratorOutMin=[]  IntegratorOutMax=[]  FilterOutMin=[]  FilterOutMax=[]  SumOutMin=[]  SumOutMax=[]  SumI1OutMin=[]  SumI1OutMax=[]  SumI2OutMin=[]  SumI2OutMax=[]  SumI3OutMin=[]  SumI3OutMax=[]  SumDOutMin=[]  SumDOutMax=[]  SaturationOutMin=[]  SaturationOutMax=[]  IntegratorContinuousStateAttributes=''  IntegratorStateMustResolveToSignalObject=off  IntegratorRTWStateStorageClass=Auto  FilterContinuousStateAttributes=''  FilterStateMustResolveToSignalObject=off  FilterRTWStateStorageClass=Auto  DifferentiatorICPrevScaledInput=0  DifferentiatorOutMin=[]  DifferentiatorOutMax=[]
  PID Controller1 : simulink/Continuous/PID Controller  Controller=PI  TimeDomain=Discrete-time  SampleTime=-1  IntegratorMethod=Backward Euler  FilterMethod=Forward Euler  Form=Parallel  UseFilter=on  ControllerParametersSource=internal  P=-0.8  I=-0.2/(60*sample_time)  D=0  N=100  InitialConditionSource=internal  InitialConditionForIntegrator=0  InitialConditionForFilter=0  ExternalReset=none  ZeroCross=off  LimitOutput=on  UpperSaturationLimit=1  LowerSaturationLimit=0  LinearizeAsGain=off  AntiWindupMode=back-calculation  Kb=1  TrackingMode=off  Kt=1  PParamMin=[]  PParamMax=[]  IParamMin=[]  IParamMax=[]  DParamMin=[]  DParamMax=[]  NParamMin=[]  NParamMax=[]  KbParamMin=[]  KbParamMax=[]  KtParamMin=[]  KtParamMax=[]  POutMin=[]  POutMax=[]  IOutMin=[]  IOutMax=[]  DOutMin=[]  DOutMax=[]  NOutMin=[]  NOutMax=[]  KbOutMin=[]  KbOutMax=[]  KtOutMin=[]  KtOutMax=[]  IntegratorOutMin=[]  IntegratorOutMax=[]  FilterOutMin=[]  FilterOutMax=[]  SumOutMin=[]  SumOutMax=[]  SumI1OutMin=[]  SumI1OutMax=[]  SumI2OutMin=[]  SumI2OutMax=[]  SumI3OutMin=[]  SumI3OutMax=[]  SumDOutMin=[]  SumDOutMax=[]  SaturationOutMin=[]  SaturationOutMax=[]  IntegratorContinuousStateAttributes=''  IntegratorStateMustResolveToSignalObject=off  IntegratorRTWStateStorageClass=Auto  FilterContinuousStateAttributes=''  FilterStateMustResolveToSignalObject=off  FilterRTWStateStorageClass=Auto  DifferentiatorICPrevScaledInput=0  DifferentiatorOutMin=[]  DifferentiatorOutMax=[]
  Saturation : Saturate  UpperLimit=1  LowerLimit=0  ZeroCross=off
  Scope{,1,3..4} (4 alike) : Scope
  Switch : Switch  Threshold=1.5
  control : Outport
  wires:
  Tcold_out/1 -> Add/1
  Add/1 -> Scope1/1, PID Controller/1, PID Controller1/1, Abs/1
  Abs/1 -> Switch/2
  PID Controller/1 -> Scope4/1, Switch/1
  PID Controller1/1 -> Switch/3, Scope3/1
  Switch/1 -> Saturation/1
  Constant/1 -> Add/2
  Saturation/1 -> control/1, Scope/1

== matlab function NatersV4_clean/Building subsystem/MATLAB Function ==
  data: Tb_in input size=[2 1]; Text input; Gin input; Psol input; Tb_out output size=[2 1]; Tws input; FH_st input; t_step parameter; time_u parameter; Qdem output size=1; T_return output
function [Tb_out, Qdem, T_return]  = Simulate_building_dynamics(Tb_in , Text, Gin, Psol, Tws, FH_st,t_step, time_u)
%#codegen
% Twr   : Return temperature of the heating system
% Tf    : Temperature of floor
% Tr    : Temperature of the room

% state matrix x = [Twr, Tf, Tin]';
% input matrix u = [Text, Tws, Gin, Psol]'
[Ab_d, Bb_d,K_fr, K_wf,K_ra, C_wr, mc_f, thermal_capacity_flow] = get_state_input_mat_building(FH_st,t_step, time_u);

% F, L,
%Tws = 35;

%Tb_out = Ab_d * Tb_in + Bb_d * [Text; Qsup; Gin; Psol];
Tb_out = Ab_d * Tb_in + Bb_d * [Text; Tws; Gin; Psol];
%Qdem = K_fr * (Tb_out(2)-Tb_out(3));

% Qdem2 = K_fr * (Tb_in(1)-Tb_in(2));
Qdem = K_ra * (Tb_in(2)-Text)-Psol-Gin;
%Qdem = K_wf * (Tb_out(1)-Tb_out(2));
%Qsup = FH_st * mc_w * (Tws-Tb_out(1));
% Qsup = K_wf * (Tb_out(1)-Tb_out(2));
% Qin = mc_f * (Tb_in(2)-Tb_out(2))/(60/time_u*60);
% test = (Qdem + Qsup) - Qin;
% e=1;
T_return = (2*K_wf*Tb_in(1) - K_wf*Tws + 2*Tws*FH_st*thermal_capacity_flow)/(K_wf + 2*FH_st*thermal_capacity_flow);

function [Ab_d, Bb_d, K_fr,K_wf,K_ra, C_wr, C_floor, thermal_capacity_flow, Qdot, facHP, nb] = get_state_input_mat_building(floor_heating_flow_fraction, t_step, time_u)

% Create the state matrix and the input matrix for the building system

% state vector for the building
% x_b = [Twr, Tf, Tin]'

% input vector for the building
% u_b = [Text, Tws, Qaux]

[C_wr, C_floor, C_room, thermal_capacity_flow, K_wf, K_fr, K_ra, Qdot] = get_param_building();

nxb = 2;
nub = 4;

A = zeros(nxb,nxb); 
B = zeros(nxb,nub); 

%L = floor_heating_flow_fraction;

%T_return = (2*K_wf*T_floor - K_wf*T_supply + 2*T_supply*floor_heating_flow_fraction*thermal_capacity_flow)/(K_wf + 2*floor_heating_flow_fraction*thermal_capacity_flow);

%% State Matrix
% Equation for temperature of the floor T_floor
A(1,1) = (K_wf^2/(C_floor*(K_wf + 2*floor_heating_flow_fraction*thermal_capacity_flow)) - (K_fr + K_wf)/C_floor);
A(1,2) = (K_fr/C_floor);

% Equation for temperature of the room T_room
A(2,1) = K_fr / C_room;
A(2,2) = - (K_fr + K_ra) / C_room;

%% Input matrix
%alpha is the Fraction of incident solar radiation on floor
alpha = 0;
% input matrix u = [Text, Tws, Gin, Psol]'
% T_floor
B(1,1) = 0;
B(1,2) = (K_wf/(2*C_floor) - (K_wf*(K_wf - 2*floor_heating_flow_fraction*thermal_capacity_flow))/(2*C_floor*(K_wf + 2*floor_heating_flow_fraction*thermal_capacity_flow)));
B(1,3) = 0;
B(1,4) = 0;
% T_room
B(2,1) = K_ra / C_room;
B(2,2) = 0;
B(2,3) = 1/C_room;
B(2,4) = (1-alpha)/C_room;

if time_u == 24
    % time_unit = 'h';
    A = A.*3600;
    B = B.*3600;
elseif time_u == 4 % 1/4h
    A = A.*60*15;
    B = B.*60*15;
elseif time_u == 12 % 5 min
    A = A.*60*5;
    B = B.*60*5;
elseif time_u == 60 % 1 min
    A = A.*60;
    B = B.*60;    
end


Ab_d = expm(t_step*A);
Bb_d = A\(Ab_d-eye(nxb))*B;


function [C_wr, mc_f, C_r, mc_w, K_wf, K_fr, K_ra, Q_D] = get_param_building()
%GET_PARAM_BUILDING returns the parameters of the selected building

cp_w = 4185;        % specific heat of water [J/kgK]
rho_w = 1000;       % density of water [kg/m3]
rho_air = 1.204;    % density of air [kg/m3]
V_w = 0.188;        % Volume of water in distribution system [m3]0.228;
V1 = 0.4;               % Volume of upper layer of storage tank [m3]
V2 = 0.4;               % Volume of middle layer of storage tank [m3]
V3 = 0.4;               % Volume of lower layer of storage tank [m3]
U_wf = 48.2;          % heat transfer coefficient of the distribution pipes [W/m2K] %48.2;
U_fr = 11.7;        % heat transfer coefficient between floor and room [W/m2K]
% \--> Source: On the heat transfer coefficients between heated/cooled radiant floorand room Tomasz Cholewaa
U_ra = 0.8;        % heat transfer coefficient of the wall [W/m2K] 1.19
A_wf = 140;         % floor heating pipes surface [m2]
A_fr = 350;         % floor surface [m2]
A_ra = 1080;         % wall surface [m2] 2*2.4H*(6l + 8L)=67.2
V_b = 6300;          % heated volume [m3]
K_wf = U_wf * A_wf; % thermal conductance of the distribution pipes [W/K]
K_fr = U_fr * A_fr; % thermal conductance between floor and room [W/K]
K_ra = U_ra * A_ra; % thermal conductance of the wall [W/K]
tau_r = 10;% 2.4
mc_f = 4.2e5;       % thermal capacity of the floor [J/K]

C_w = cp_w * rho_w * (V_w);%+V1+V2+V3);   % thermal capacity water [J/K]
%C_r = K_ra * tau_r;         % thermal capacity of the room [J/K]
C_r = V_b * rho_air * 1005 * tau_r; % thermal capacity of the room [J/K]
% Design hydronic system, rules Karlsson_and_Fahlen_2008
Text_D = -10;                   % Design outdoor temperature [K] 
Tin_D = 20;                     % Design outdoor temperature [K] 
Ts_D = 35;                      % Design supply temperature [K]  
Tr_D = 28;                      % Design return temperature [K]
Q_D = K_ra * (Tin_D - Text_D);  % Design heat demand [W]
mc_w = Q_D / (Ts_D - Tr_D);     % Design thermal capacity flow [W/K]
tau_HP =3*60;                   % Time constant Heat Pump [s]
C_ws = tau_HP * mc_w;           % thermal capacity supply water [J/K]
C_wr = (C_w - C_ws);        % thermal capacity return water [J/K]
